simulink model "ejercicio5"  (R2024b)
settings: Solver=VariableStepAuto  StartTime=0.0  StopTime=5  RelTol=1e-3
settings Model: Creator=david.andrino  LastModifiedBy=Ruben
settings DataIOCC: ReturnWorkspaceOutputs=off
settings RTWCC: GPUComputeCapability=3.5

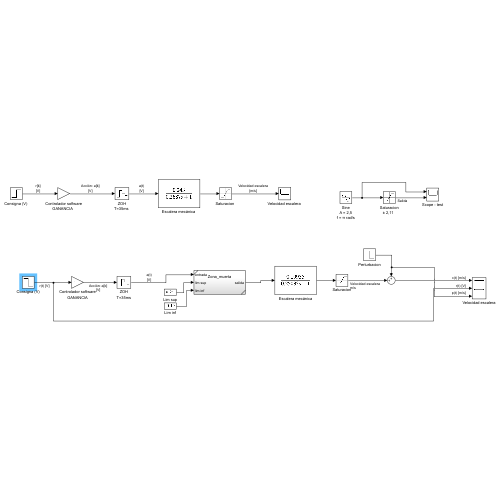
[thumbnail: Simulink's stored preview of the top-level diagram]
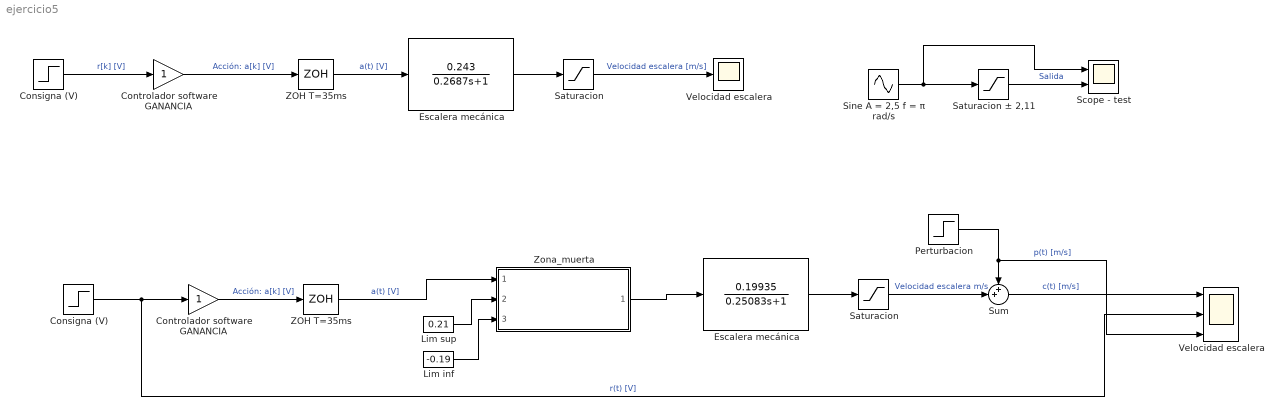
== system ejercicio5 ==
  Consigna (V) : Step  Time=0  After=-1  SampleTime=0
  "Consigna (V) " : Step  Time=0  After=20  SampleTime=0
  Controlador software GANANCIA : Gain
  "Controlador software GANANCIA  " : Gain
  Escalera mecánica : TransferFcn  Numerator=0.19935  Denominator=[0.25083 1]
  "Escalera mecánica " : TransferFcn  Numerator=0.243  Denominator=[0.2687 1]
  Lim inf : Constant  Value=-0.19
  Lim sup : Constant  Value=0.21
  Perturbacion : Step  Time=2.5  After=-0.1  SampleTime=0
  Saturacion : Saturate  UpperLimit=2.11  LowerLimit=-2.11
  "Saturacion ± 2,11  " : Saturate  UpperLimit=2.11  LowerLimit=-2.11
  "Saturacion " : Saturate  UpperLimit=2000  LowerLimit=-2.11
  Scope - test : Scope  NumInputPorts=2
  Sine A = 2,5 f = π rad/s : Sin  Amplitude=2.5  Frequency=pi  SampleTime=0
  Sum : Sum  Inputs=++|
  Velocidad escalera : Scope  NumInputPorts=3
  "Velocidad escalera " : Scope
  ZOH T=35ms : ZeroOrderHold  SampleTime=35e-3
  "ZOH T=35ms " : ZeroOrderHold  SampleTime=35e-3
  Zona_muerta : Subsystem  ReferencedSubsystem=Zona_muerta
  wires:
  Consigna (V)/1 -> Controlador software GANANCIA/1, Velocidad escalera/2  "r(t) [V]"
  Controlador software GANANCIA/1 -> ZOH T=35ms/1  "Acción: a[k] [V]"
  Zona_muerta/1 -> Escalera mecánica/1
  Escalera mecánica/1 -> Saturacion/1
  "Escalera mecánica "/1 -> "Saturacion "/1
  "Saturacion "/1 -> "Velocidad escalera "/1  "Velocidad escalera [m/s]"
  "ZOH T=35ms "/1 -> "Escalera mecánica "/1  "a(t) [V]"
  "Controlador software GANANCIA  "/1 -> "ZOH T=35ms "/1  "Acción: a[k] [V]"
  "Consigna (V) "/1 -> "Controlador software GANANCIA  "/1  "r[k] [V]"
  "Saturacion ± 2,11  "/1 -> Scope - test/2  "Salida"
  Sine A = 2,5 f = π rad/s/1 -> Scope - test/1, "Saturacion ± 2,11  "/1
  ZOH T=35ms/1 -> Zona_muerta/1  "a(t) [V]"
  Lim sup/1 -> Zona_muerta/2
  Lim inf/1 -> Zona_muerta/3
  Sum/1 -> Velocidad escalera/1  "c(t) [m/s]"
  Perturbacion/1 -> Velocidad escalera/3, Sum/1  "p(t) [m/s]"
  Saturacion/1 -> Sum/2  "Velocidad escalera m/s"
